simulink subsystem "Generator_V2"  (R2024a)
settings: Solver=VariableStepAuto  StartTime=0.0  StopTime=10.0  RelTol=1e-3
PreLoadFcn:
  | k_e = 5.4e-3;
  | R_a = 1.94e-3;
  | L = 77e-6;
undefined symbols (not defined in the file): Ke, Ls, magnitude, P, Ra
settings Model: Creator=User  LastModifiedBy=Henrique Mesquita

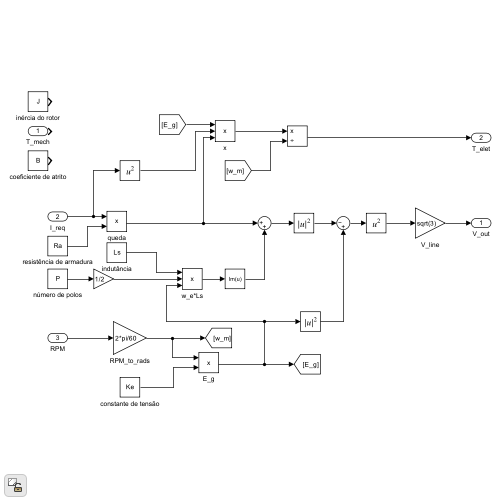
[thumbnail: Simulink's stored preview of the top-level diagram]
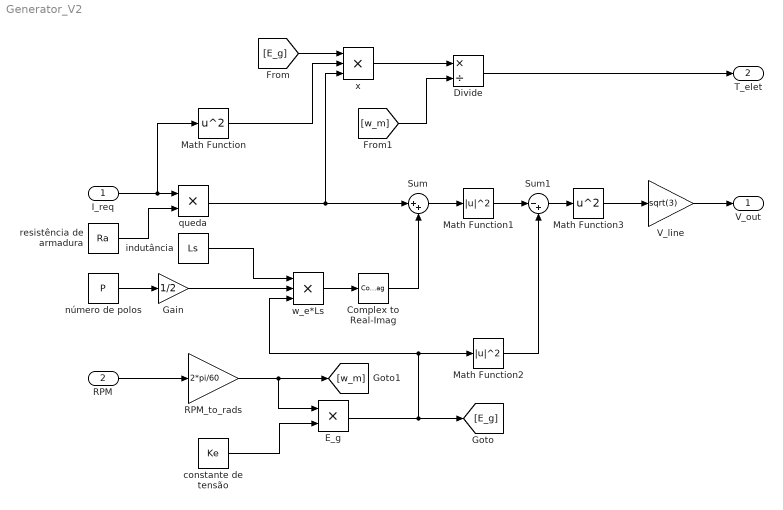
== system Generator_V2 ==
  I_req : Inport
  RPM : Inport  Port=2
  Complex to Real-Imag : ComplexToRealImag  Output=Imag
  Divide : Product  Inputs=*/
  E_g : Product  Inputs=**
  Gain : Gain  Gain=1/2
  Math Function : Math  Operator=square
  Math Function1 : Math  Operator=magnitude^2
  Math Function2 : Math  Operator=magnitude^2
  Math Function3 : Math  Operator=square
  RPM_to_rads : Gain  Gain=2*pi/60
  Sum : Sum  Inputs=|++
  Sum1 : Sum  Inputs=|-+
  V_line : Gain  Gain=sqrt(3)
  constante de tensão : Constant  Value=Ke
  indutância : Constant  Value=Ls
  número de polos : Constant  Value=P
  queda : Product  Inputs=**
  resistência de armadura : Constant  Value=Ra
  w_e*Ls : Product  Inputs=***
  x : Product  Inputs=***
  V_out : Outport
  T_elet : Outport  Port=2
  wires:
  RPM/1 -> RPM_to_rads/1
  RPM_to_rads/1 -> [w_m], E_g/1
  constante de tensão/1 -> E_g/2
  número de polos/1 -> Gain/1
  E_g/1 -> [E_g], Math Function2/1, w_e*Ls/3
  I_req/1 -> Math Function/1, queda/1
  resistência de armadura/1 -> queda/2
  Sum1/1 -> Math Function3/1
  V_line/1 -> V_out/1
  Gain/1 -> w_e*Ls/2
  indutância/1 -> w_e*Ls/1
  queda/1 -> x/3, Sum/1
  Sum/1 -> Math Function1/1
  w_e*Ls/1 -> Complex to Real-Imag/1
  Complex to Real-Imag/1 -> Sum/2
  [E_g] -> x/1
  Math Function/1 -> x/2
  x/1 -> Divide/1
  [w_m] -> Divide/2
  Divide/1 -> T_elet/1
  Math Function1/1 -> Sum1/1
  Math Function2/1 -> Sum1/2
  Math Function3/1 -> V_line/1
